simulink model "sloworbcorr_ps_voltage"  (Simulink 7.8)
settings: Solver=ode45  StartTime=0.0  StopTime=10.0  RelTol=1e-3
values from neighbouring files (symbols this model uses):
  corrsofbpsfilter = param.corrsofbpsfilter    [simfofb.m]
settings Model: Creator=danielot  LastModifiedBy=danielot

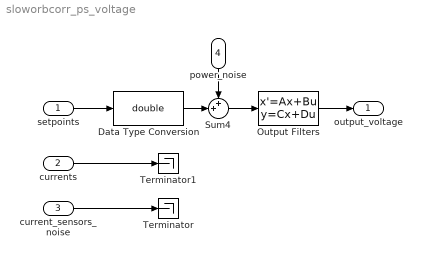
== system sloworbcorr_ps_voltage ==
  setpoints : Inport  PortDimensions=ncorrsofb
  currents : Inport  Port=2  PortDimensions=ncorrsofb
  current_sensors_noise : Inport  Port=3  PortDimensions=ncorrsofb
  power_noise : Inport  Port=4
  Data Type Conversion : DataTypeConversion  OutDataTypeStr=double
  Output Filters : StateSpace  A=corrsofbpsfilter.a  B=corrsofbpsfilter.b  C=corrsofbpsfilter.c  D=corrsofbpsfilter.d
  Sum4 : Sum  Inputs=++|
  Terminator : Terminator
  Terminator1 : Terminator
  output_voltage : Outport
  wires:
  power_noise/1 -> Sum4/1
  Output Filters/1 -> output_voltage/1
  Sum4/1 -> Output Filters/1
  setpoints/1 -> Data Type Conversion/1
  Data Type Conversion/1 -> Sum4/2
  current_sensors_noise/1 -> Terminator/1
  currents/1 -> Terminator1/1
